simulink model "SPWM_Inverter"  (Simulink 7.5)
settings: Solver=ode23  StartTime=0.0  StopTime=5  MaxStep=0.0001  RelTol=1e-3
libraries: powerlib x10, simulink x1
settings Model: Creator=lm  LastModifiedBy=lm

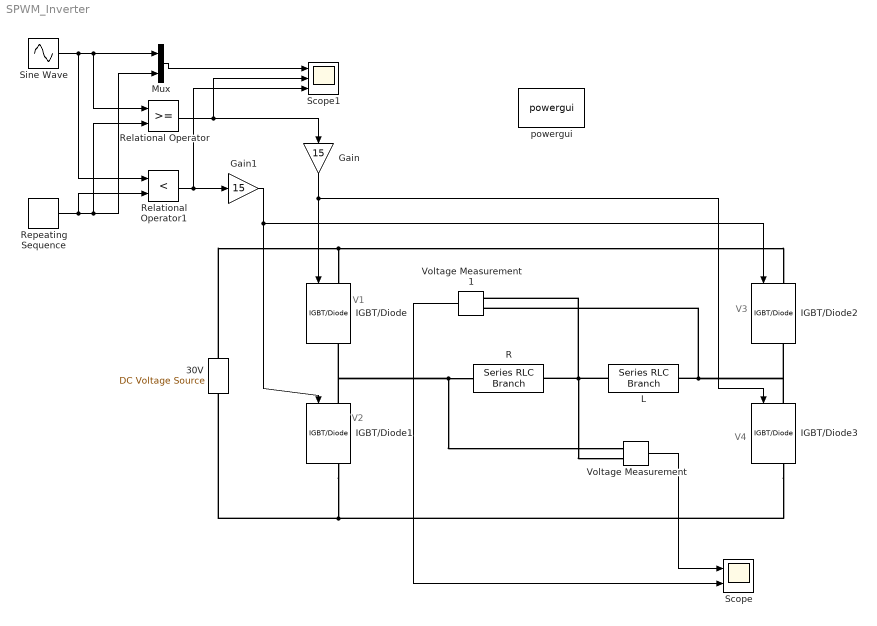
== system SPWM_Inverter ==
  note: V1
  note: V2
  note: V4
  note: V3
  30V : powerlib/Electrical Sources/DC Voltage Source  DialogController=POWERSYS.PowerSysDialog  SystemSampleTime=-1  Amplitude=30  Measurements=None
  Gain : Gain  Gain=15  ParameterDataType=fixdt(1, 16)  ParameterScaling=2^0  OutDataType=fixdt(1, 16)  OutScaling=2^0
  Gain1 : Gain  Gain=15  ParameterDataType=fixdt(1, 16)  ParameterScaling=2^0  OutDataType=fixdt(1, 16)  OutScaling=2^0
  IGBT/Diode{,1..3} (4 alike) : powerlib/Power Electronics/IGBT//Diode  DialogController=POWERSYS.PowerSysDialog  SystemSampleTime=-1  Ron=1e-3  Rs=1e5  Cs=inf  Measurements=on
  L : powerlib/Elements/Series RLC Branch  DialogController=POWERSYS.PowerSysDialog  PhysicalDomain=powersysdomain  SubClassName=unknown  LeftPortType=p1  RightPortType=p1  LConnTagsString=__new0  RConnTagsString=__new0  BranchType=L  Resistance=1e-5  Inductance=1e-2  SetiL0=off  InitialCurrent=0  Capacitance=1e-6  Setx0=off  InitialVoltage=0  Measurements=None
  Mux : Mux  Inputs=2
  R : powerlib/Elements/Series RLC Branch  DialogController=POWERSYS.PowerSysDialog  PhysicalDomain=powersysdomain  SubClassName=unknown  LeftPortType=p1  RightPortType=p1  LConnTagsString=__new0  RConnTagsString=__new0  BranchType=R  Resistance=40  Inductance=1e-3  SetiL0=off  InitialCurrent=0  Capacitance=1e-6  Setx0=off  InitialVoltage=0  Measurements=Branch voltage
  Relational Operator : RelationalOperator  LogicOutDataTypeMode=boolean  LogicDataType=fixdt(0, 8)  OutDataTypeStr=boolean
  Relational Operator1 : RelationalOperator  Operator=<  LogicOutDataTypeMode=boolean  LogicDataType=fixdt(0, 8)  OutDataTypeStr=boolean
  Repeating Sequence : simulink/Sources/Repeating Sequence  SystemSampleTime=-1  rep_seq_t=[0 0.01]  rep_seq_y=[-1 1]
  Scope : Scope  NumInputPorts=2
      settings: TimeRange=0.2  YMin=-80~-5  YMax=80~5  SaveName=voltage
  Scope1 : Scope  NumInputPorts=3
      settings: YMin=-5~-5~-5  YMax=5~5~5
  Sine Wave : Sin  Amplitude=0.95  Bias=0  Frequency=3000/(2*pi)  Phase=0  Samples=10  SampleTime=0  Offset=0
  Voltage Measurement : powerlib/Measurements/Voltage Measurement  DialogController=POWERSYS.PowerSysDialog  SystemSampleTime=-1  PhasorSimulation=off  OutputType=Complex  PSBequivalent=0
  Voltage Measurement1 : powerlib/Measurements/Voltage Measurement  DialogController=POWERSYS.PowerSysDialog  SystemSampleTime=-1  PhasorSimulation=off  OutputType=Complex  PSBequivalent=0
  powergui : powerlib/powergui  Priority=1  SystemSampleTime=-1  SimulationMode=Discrete  SampleTime=50e-6  frequency=60  SPID=off  DisableSnubberDevices=off  DisableRonSwitches=off  DisableVfSwitches=off  SwTol=0  Interpol=off  frequencyindice=0  echomessages=off  HookPort=off  DisplayEquations=off  FunctionMessages=off  EnableUseOfTLC=off  x0status=blocks  RestoreLinks=warning  ResistiveCurrentMeasurement=off  Ylog=off  Xlog=on  ShowGrid=off  save=off  variable=ZData  structure=voltage  ZoomFFT=on  StartTime=0.0  cycles=1  DisplayStyle=1  fundamental=100  FreqAxis=off  MaxFrequency=1000  frequencyindicesteady=1  display=off  methode=off
  wires:
  Sine Wave/1 -> Mux/1, Relational Operator/1, Relational Operator1/1
  Repeating Sequence/1 -> Mux/2, Relational Operator/2, Relational Operator1/2
  Relational Operator/1 -> Scope1/2, Gain/1
  Relational Operator1/1 -> Scope1/3, Gain1/1
  Mux/1 -> Scope1/1
  Voltage Measurement/1 -> Scope/1
  Voltage Measurement1/1 -> Scope/2
  Gain1/1 -> IGBT/Diode1/1, IGBT/Diode2/1
  Gain/1 -> IGBT/Diode/1, IGBT/Diode3/1
  connections:
  IGBT/Diode1/LConn1 -- IGBT/Diode/RConn1 -- R/RConn1 -- Voltage Measurement/LConn1
  IGBT/Diode1/RConn1 -- 30V/LConn1 -- IGBT/Diode3/RConn1
  30V/RConn1 -- IGBT/Diode/LConn1 -- IGBT/Diode2/LConn1
  Voltage Measurement/LConn2 -- L/LConn1 -- R/LConn1 -- Voltage Measurement1/LConn1
  IGBT/Diode3/LConn1 -- IGBT/Diode2/RConn1 -- L/RConn1 -- Voltage Measurement1/LConn2
